simulink model "Control_Model_v3_1"  (R2015a)
settings: Solver=ode1  StartTime=0.0  StopTime=40  FixedStep=0.002  MaxStep=0.01  MinStep=0.01  RelTol=1e-3
settings Model: Creator=Callum  LastModifiedBy=Callum
settings SolverCC: InitialStep=0.01
settings HardwareCC: TargetLongLongMode=on  TargetIntDivRoundTo=Zero  TargetEndianess=LittleEndian  TargetHWDeviceType=MATLAB Host  ProdEqTarget=off
settings RTWCC: SystemTargetFile=rsim.tlc  TemplateMakefile=rsim_default_tmf  Description=Rapid Simulation Target
settings RSimTargetCC: ERTMultiwordTypeDef=System defined  ERTMultiwordLength=256

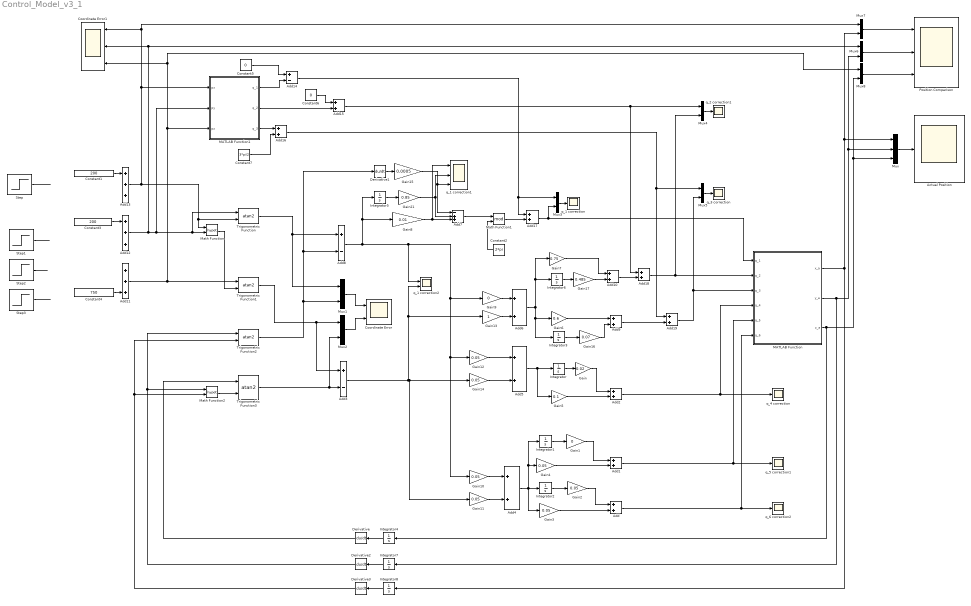
== system Control_Model_v3_1 ==
  Actual Position : Scope
      settings: YMin=-400  YMax=1200
  Add{,1..2,4..6,9..10,15..19} (13 alike) : Sum
  Add11 : Sum  Inputs=+++
  Add12 : Sum  Inputs=+++
  Add13 : Sum  Inputs=+++
  Add14 : Sum  Inputs=+-
  Add3 : Sum  Inputs=+-
  Add7 : Sum  Inputs=-++
  Add8 : Sum  Inputs=+-
  Constant1 : Constant  Value=200
  Constant2 : Constant  Value=2*pi
  Constant3 : Constant  Value=200
  Constant4 : Constant  Value=750
  Constant5 : Constant  Value=0
  Constant6 : Constant  Value=0
  Constant7 : Constant  Value=3*pi/2
  Coordinate Error : Scope  NumInputPorts=2
      settings: YMin=-5~-5  YMax=5~5  SaveName=error
  Coordinate Error1 : Scope  NumInputPorts=3
      settings: YMin=-5~-5~-5  YMax=5~5~5  SaveName=ScopeData10
  Derivative{,1..3} (4 alike) : Derivative
  Gain : Gain  Gain=0.02
  Gain1 : Gain  Gain=0
  Gain{2..4,10..12,14} (7 alike) : Gain  Gain=0.05
  Gain13 : Gain
  Gain15 : Gain  Gain=0.0005
  Gain16 : Gain  Gain=0.07
  Gain17 : Gain  Gain=0.485
  Gain21 : Gain  Gain=0.85
  Gain5 : Gain  Gain=0.1
  Gain6 : Gain  Gain=0.6
  Gain7 : Gain  Gain=0.75
  Gain8 : Gain  Gain=0.01
  Gain9 : Gain  Gain=0
  Integrator{,1..8} (9 alike) : Integrator
  MATLAB Function : MATLAB Function  TreatAsAtomicUnit=on
  MATLAB Function1 : MATLAB Function  TreatAsAtomicUnit=on
  Math Function : Math  Operator=hypot  SaturateOnIntegerOverflow=on
  Math Function1 : Math  Operator=mod  SaturateOnIntegerOverflow=on
  Math Function2 : Math  Operator=hypot  SaturateOnIntegerOverflow=on
  Mux : Mux  Inputs=3
  Mux{1..8} (8 alike) : Mux  Inputs=2
  Position Comparison : Scope  NumInputPorts=3
      settings: YMin=-400~-5~-5  YMax=1200~5~5  SaveName=Position
  Step : Step  After=-60  SampleTime=0
  Step1 : Step  After=-50  SampleTime=0
  Step2 : Step  After=0  SampleTime=0
  Step3 : Step  After=100  SampleTime=0
  Trigonometric Function{,1..3} (4 alike) : Trigonometry  Operator=atan2
  q_1 correction : Scope
      settings: TimeRange=20  YMin=0  YMax=6.5
  q_1 correction1 : Scope  NumInputPorts=3
      settings: YMin=-5~-5~-5  YMax=5~5~5  SaveName=ScopeData5
  q_1 correction2 : Scope  NumInputPorts=2
      settings: YMin=-5~-5  YMax=5~5  SaveName=ScopeData6
  q_2 correction1 : Scope
      settings: SaveName=ScopeData2
  q_3 correction : Scope
      settings: SaveName=ScopeData3
  q_4 correction : Scope
      settings: SaveName=ScopeData4
  q_5 correction1 : Scope
      settings: SaveName=ScopeData12
  q_6 correction2 : Scope
      settings: SaveName=ScopeData13
  wires:
  Integrator/1 -> Gain/1
  Integrator1/1 -> Gain1/1
  Integrator2/1 -> Gain2/1
  Gain2/1 -> Add/1
  Gain3/1 -> Add/2
  Add/1 -> MATLAB Function/6(q_6), q_6 correction2/1
  Gain1/1 -> Add1/1
  Add1/1 -> MATLAB Function/5(q_5), q_5 correction1/1
  Gain4/1 -> Add1/2
  Add2/1 -> MATLAB Function/4(q_4), q_4 correction/1
  Gain/1 -> Add2/1
  Gain5/1 -> Add2/2
  Add5/1 -> Gain5/1, Integrator/1
  Add6/1 -> Integrator3/1, Gain6/1, Integrator6/1, Gain7/1
  Add11/1 -> Mux8/1, Coordinate Error1/3, MATLAB Function1/3(pz), Trigonometric Function1/1
  MATLAB Function/1(x_a) -> Integrator8/1, Mux/1, Mux7/2
  Gain10/1 -> Add4/1
  Gain14/1 -> Add5/2
  Gain6/1 -> Add9/1
  Derivative/1 -> Trigonometric Function3/1
  Integrator5/1 -> Gain21/1
  Gain21/1 -> q_1 correction1/2, Add7/2
  Add7/1 -> Math Function1/1
  Gain8/1 -> q_1 correction1/1, Add7/3
  Gain12/1 -> Add5/1
  Gain13/1 -> Add6/2
  Gain9/1 -> Add6/1
  Add3/1 -> Gain11/1, Gain14/1, Gain13/1, q_1 correction2/2
  Math Function/1 -> Trigonometric Function1/2
  Derivative1/1 -> Gain15/1
  Gain15/1 -> Add7/1, q_1 correction1/3
  Constant2/1 -> Math Function1/2
  Integrator3/1 -> Gain16/1
  Gain16/1 -> Add9/2
  Integrator6/1 -> Gain17/1
  Gain7/1 -> Add10/1
  Gain17/1 -> Add10/2
  Integrator8/1 -> Derivative3/1
  Derivative3/1 -> Math Function2/2, Trigonometric Function2/2
  Mux/1 -> Actual Position/1
  Mux1/1 -> Coordinate Error/1
  Derivative2/1 -> Math Function2/1, Trigonometric Function2/1
  Trigonometric Function/1 -> Add8/1, Mux1/1
  Trigonometric Function2/1 -> Add8/2, Derivative1/1, Mux1/2
  Math Function2/1 -> Trigonometric Function3/2
  Trigonometric Function3/1 -> Mux2/2, Add3/2
  Trigonometric Function1/1 -> Add3/1, Mux2/1
  Mux2/1 -> Coordinate Error/2
  Integrator4/1 -> Derivative/1
  MATLAB Function/3(z_a) -> Integrator4/1, Mux/3, Mux8/2
  Integrator7/1 -> Derivative2/1
  Add8/1 -> Gain9/1, Gain12/1, Gain10/1, q_1 correction2/1, Integrator5/1, Gain8/1
  Step2/1 -> ?
  Step3/1 -> ?
  Constant4/1 -> Add11/3
  Step1/1 -> ?
  Constant3/1 -> Add12/1
  Step/1 -> ?
  Constant1/1 -> Add13/1
  MATLAB Function1/1(q_1) -> Add14/2
  Constant5/1 -> Add14/1
  MATLAB Function1/2(q_2) -> Add15/2
  Constant6/1 -> Add15/1
  MATLAB Function1/3(q_3) -> Add16/1
  Constant7/1 -> Add16/2
  Add14/1 -> Add17/1, Mux3/1
  Add16/1 -> Mux5/1, Add19/1
  Math Function1/1 -> Add17/2
  Add17/1 -> Mux3/2, MATLAB Function/1(q_1)
  Add18/1 -> MATLAB Function/2(q_2), Mux4/2
  Add10/1 -> Add18/2
  Add9/1 -> Add19/2
  Add19/1 -> MATLAB Function/3(q_3), Mux5/2
  Mux3/1 -> q_1 correction/1
  Mux4/1 -> q_2 correction1/1
  Mux5/1 -> q_3 correction/1
  Add15/1 -> Add18/1, Mux4/1
  Add13/1 -> Mux7/1, Coordinate Error1/1, MATLAB Function1/1(px), Trigonometric Function/2, Math Function/1
  Mux7/1 -> Position Comparison/1
  MATLAB Function/2(y_a) -> Integrator7/1, Mux/2, Mux6/2
  Add12/1 -> Math Function/2, Trigonometric Function/1, MATLAB Function1/2(py), Mux6/1, Coordinate Error1/2
  Mux6/1 -> Position Comparison/2
  Mux8/1 -> Position Comparison/3
  Gain11/1 -> Add4/2
  Add4/1 -> Gain3/1, Integrator1/1, Gain4/1, Integrator2/1

== matlab function Control_Model_v3_1/MATLAB Function1 ==
  data: px input; py input; pz input; q_1 output; q_2 output; q_3 output
function [q_1, q_2, q_3] = fcn( px, py, pz)
%#codegen

D1 = 197.13;%275.5;
D2 = 410;
D3 = 207.3;
D4 = 74.1;
D5 = 74.1;
D6 = 160.0;
e2 = 9.8;
d1 = 197.13;
d2 = D2;
d3 = D3;

% q_3 +
%q_3__ = 1 * acos( (px^2 + (pz-d1)^2 - d2^2 - d3^2) / (2*d2*d3) );  

%cq_2 = (px*(d2+d3*cos(q_3__)) + d3*sin(q_3__)*(pz -d1)) / (d2^2 + d3^2 + 2*d2*d3*cos(q_3__));
%sq_2 = (-px*d3*sin(q_3__) + (d2+d3*cos(q_3__))*(pz -d1)) / (d2^2 + d3^2 + 2*d2*d3*cos(q_3__));
%q_2__ = (pi/2) - atan2(sq_2,cq_2);
%q_3__*180/pi
%q_2__*180/pi
% q_3 -

q_3 = 1 * acos( (px^2 + (pz-d1)^2 - d2^2 - d3^2) / (2*d2*d3) );  

cq_2 = (px*(d2+d3*cos(q_3)) + d3*sin(q_3)*(pz -d1)) / (d2^2 + d3^2 + 2*d2*d3*cos(q_3));
sq_2 = (-px*d3*sin(q_3) + (d2+d3*cos(q_3))*(pz -d1)) / (d2^2 + d3^2 + 2*d2*d3*cos(q_3));
q_2 = (pi/2) - atan2(sq_2,cq_2);

% q_1 offset
q_1 = atan2((py), px) - asin(e2 / ((px^2 + py^2)^.5));

== matlab function Control_Model_v3_1/MATLAB Function ==
  data: q_1 input; x_a output; q_2 input; q_3 input; q_4 input; q_5 input; q_6 input; y_a output; z_a output
function [x_a, y_a, z_a] = fcn(q_1, q_2, q_3, q_4, q_5, q_6)
%#codegen

q1 = q_1;%pi-(q_1);
q2 = q_2;%-pi/2 + (q_2+pi);
q3 = q_3;%pi/2 + (pi+q_3);
q4 = q_4;%q_4;
q5 = q_5;%-pi + q_5;
q6 = q_6;%pi + q_6;

%A_new = vpa(subs(A, [q1,q2,q3,q4,q5,q6], [ pi-(q_1), -pi/2 + (q_2+pi), pi/2 + (pi+q_3), q_4, -pi + q_5, pi]));


x_a = 9.8*sin(q1) + 410.0*cos(q1)*cos(q2) - 161.90703230275506147226218323136*cos(q4)*sin(q1) + 175.614064605510166451876962007*sin(q5)*(1.0*sin(q1)*sin(q4) - cos(q4)*(cos(q1)*cos(q2)*cos(q3) + cos(q1)*sin(q2)*sin(q3))) - 161.90703230275506147226218323136*sin(q4)*(cos(q1)*cos(q2)*cos(q3) + cos(q1)*sin(q2)*sin(q3)) - 175.614064605510166451876962007*cos(q5)*(0.5*cos(q4)*sin(q1) + 0.5*sin(q4)*(cos(q1)*cos(q2)*cos(q3) + cos(q1)*sin(q2)*sin(q3)) - 0.86602540378443864676372317075294*cos(q1)*cos(q2)*sin(q3) + 0.86602540378443864676372317075294*cos(q1)*cos(q3)*sin(q2)) - 343.55872363064032981583295622841*cos(q1)*cos(q2)*sin(q3) + 343.55872363064032981583295622841*cos(q1)*cos(q3)*sin(q2); 
y_a = 161.90703230275506147226218323136*cos(q1)*cos(q4) - 9.8*cos(q1) + 410.0*cos(q2)*sin(q1) + 175.614064605510166451876962007*cos(q5)*(0.5*cos(q1)*cos(q4) - 0.5*sin(q4)*(sin(q1)*sin(q2)*sin(q3) + cos(q2)*cos(q3)*sin(q1)) + 0.86602540378443864676372317075294*cos(q2)*sin(q1)*sin(q3) - 0.86602540378443864676372317075294*cos(q3)*sin(q1)*sin(q2)) - 175.614064605510166451876962007*sin(q5)*(1.0*cos(q1)*sin(q4) + cos(q4)*(sin(q1)*sin(q2)*sin(q3) + cos(q2)*cos(q3)*sin(q1))) - 161.90703230275506147226218323136*sin(q4)*(sin(q1)*sin(q2)*sin(q3) + cos(q2)*cos(q3)*sin(q1)) - 343.55872363064032981583295622841*cos(q2)*sin(q1)*sin(q3) + 343.55872363064032981583295622841*cos(q3)*sin(q1)*sin(q2);
z_a = 410.0*sin(q2) - 343.55872363064032981583295622841*cos(q2)*cos(q3) - 343.55872363064032981583295622841*sin(q2)*sin(q3) + 175.614064605510166451876962007*cos(q5)*(0.86602540378443864676372317075294*cos(q2)*cos(q3) + 0.86602540378443864676372317075294*sin(q2)*sin(q3) + 0.5*sin(q4)*(1.0*cos(q2)*sin(q3) - 1.0*cos(q3)*sin(q2))) + 161.90703230275506147226218323136*sin(q4)*(1.0*cos(q2)*sin(q3) - 1.0*cos(q3)*sin(q2)) + 175.614064605510166451876962007*cos(q4)*sin(q5)*(1.0*cos(q2)*sin(q3) - 1.0*cos(q3)*sin(q2)) + 197.13;




%y = u;
